simulink model "monoaxial_AZ"  (R2023b)
settings: Solver=VariableStepAuto  StartTime=0.0  StopTime=50  RelTol=1e-3
values from neighbouring files (symbols this model uses):
  meas_noise = 0.0001    [monoaxial_AZ.m]
  poles = pole(Gz)    [monoaxial_AZ.m]
  sat = 1.2    [monoaxial_AZ.m]
  Ts = 0.05    [monoaxial_AZ.m]
libraries: simulink x2, slpidlib x1
settings Model: Creator=alexz  LastModifiedBy=alexz

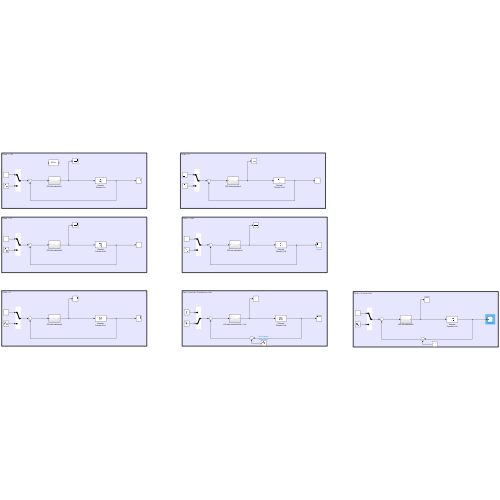
[thumbnail: Simulink's stored preview of the top-level diagram]
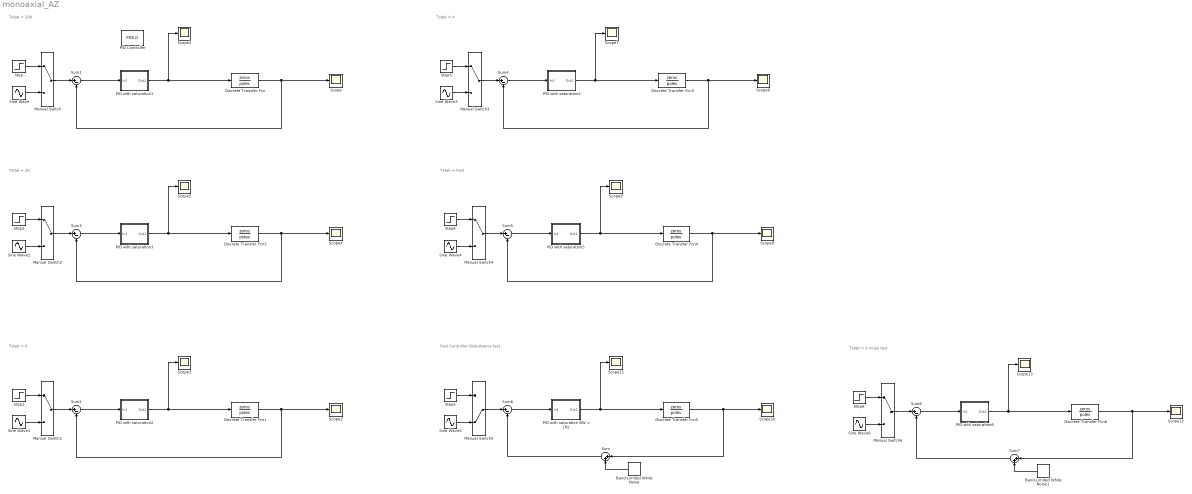
== system monoaxial_AZ ==
  note: Tstab = 100
  note: Tstab = 6
  note: Tstab = 20
  note: Tstab = 4
  note: Tstab = Fast
  note: Fast Controller Disturbance test
  note: Tstab = 4 noise test
  Band-Limited White Noise : simulink/Sources/Band-Limited White Noise  Cov=[meas_noise]  Ts=0.05  seed=[23341]
  Band-Limited White Noise1 : simulink/Sources/Band-Limited White Noise  Cov=[meas_noise]  Ts=0.05  seed=[23341]
  Discrete Transfer Fcn{,1..6} (7 alike) : DiscreteTransferFcn  Numerator=zeros  Denominator=poles
  Manual Switch{,1..4,6} (6 alike) : ManualSwitch
  Manual Switch5 : ManualSwitch  CurrentSetting=0
  PID Controller : slpidlib/PID Controller  Controller=PID  Form=Parallel  TimeDomain=Discrete-time  UseExternalTs=off  SampleTime=-1  IntegratorMethod=Forward Euler  FilterMethod=Forward Euler  ControllerParametersSource=internal  P=-0.0499947918294246  I=-1.99979167317699  UseKiTs=off  D=0  N=100  UseFilter=on  TunerSelectOption=Transfer Function Based (PID Tuner App)  InitialConditionSource=internal  InitialConditionForIntegrator=0  InitialConditionForFilter=0  DifferentiatorICPrevScaledInput=0  ExternalReset=none  TrackingMode=off  Kt=1  LimitOutput=off  SatLimitsSource=internal  UpperSaturationLimit=inf  LowerSaturationLimit=-inf  LinearizeAsGain=on  AntiWindupMode=none  Kb=1  LimitIntegrator=off  UpperIntegratorSaturationLimit=inf  LowerIntegratorSaturationLimit=-inf  POutMin=[]  POutMax=[]  IOutMin=[]  IOutMax=[]  DOutMin=[]  DOutMax=[]  NOutMin=[]  NOutMax=[]  SumOutMin=[]  SumOutMax=[]  SaturationOutMin=[]  SaturationOutMax=[]  PParamMin=[]  PParamMax=[]  IParamMin=[]  IParamMax=[]  DParamMin=[]  DParamMax=[]  NParamMin=[]  NParamMax=[]  KbParamMin=[]  KbParamMax=[]  KtParamMin=[]  KtParamMax=[]  KbOutMin=[]  KbOutMax=[]  KtOutMin=[]  KtOutMax=[]  IntegratorOutMin=[]  IntegratorOutMax=[]  FilterOutMin=[]  FilterOutMax=[]  SumI1OutMin=[]  SumI1OutMax=[]  SumI2OutMin=[]  SumI2OutMax=[]  SumI3OutMin=[]  SumI3OutMax=[]  SumI4OutMin=[]  SumI4OutMax=[]  SumDOutMin=[]  SumDOutMax=[]  DifferentiatorOutMin=[]  DifferentiatorOutMax=[]  FilterDiffOutCoefMin=[]  FilterDiffOutCoefMax=[]  ReciprocalOutMin=[]  ReciprocalOutMax=[]  SumDenOutMin=[]  SumDenOutMax=[]  SumNumOutMin=[]  SumNumOutMax=[]  DivideOutMin=[]  DivideOutMax=[]  UdiffTsProdOutMin=[]  UdiffTsProdOutMax=[]  NTsProdOutMin=[]  NTsProdOutMax=[]  UintegralTsProdOutMin=[]  UintegralTsProdOutMax=[]  UngainTsProdOutMin=[]  UngainTsProdOutMax=[]  ClampingZeroOutDataTypeStr=Inherit: Inherit via back propagation  ClampingZeroOutMin=[]  ClampingZeroOutMax=[]  FilterDenConstantOutDataTypeStr=Inherit: Inherit via back propagation  FilterDenConstantOutMin=[]  FilterDenConstantOutMax=[]  PCopyOutDataTypeStr=Inherit: Inherit via back propagation  PCopyOutMin=[]  PCopyOutMax=[]  NCopyOutDataTypeStr=Inherit: Inherit via back propagation  NCopyOutMin=[]  NCopyOutMax=[]  IntegratorContinuousStateAttributes=''  IntegratorStateMustResolveToSignalObject=off  IntegratorRTWStateStorageClass=Auto  FilterContinuousStateAttributes=''  FilterStateMustResolveToSignalObject=off  FilterRTWStateStorageClass=Auto  ParallelPVariant=InternalParameters  IdealPVariant=Disabled  IVariant=InternalParameters  DVariant=InternalParameters  IntegratorVariant=Discrete  SatVariant=Disabled  AWVariant=Passthrough  PCopyVariant=Disabled  TRVariant=Disabled  FdbkBlocksVariant=Forward  IdealPFdbkVariant=Disabled  SatFdbkVariant=Disabled  DerivativeFilterVariant=ForwardEulerFilter  NVariant=InternalParameters  NCopyVariant=Disabled  FilterICVariant=InternalICsFilter  IntegratorICVariant=InternalICs  ExternalResetVariant=Disabled  TRSumVariant=Passthrough  SumFdbkVariant=Disabled  SumVariant=Sum_PID  TsampFilterVariant=InternalTs  TsampNgainVariant=Passthrough  TsampIntegralVariant=Disabled_SignalSpec  ExternalSaturationOutDataTypeStr=Inherit: Same as second input
  PID with saturation BW = 1Hz : Subsystem
  PID with saturation1 : Subsystem
  PID with saturation2 : Subsystem
  PID with saturation3 : Subsystem
  PID with saturation4 : Subsystem
  PID with saturation5 : Subsystem
  PID with saturation6 : Subsystem
  Scope{,1..13} (14 alike) : Scope
  Sine Wave : Sin  SampleTime=0.05
  Sine Wave{1,3..6} (5 alike) : Sin  Amplitude=0.5  Frequency=0.1  SampleTime=0.05
  Sine Wave2 : Sin  SampleTime=0.05
  Step{,1..6} (7 alike) : Step  After=0.5  SampleTime=0.05
  Sum : Sum  Inputs=|++
  Sum{1..6,8} (7 alike) : Sum  Inputs=|+-
  Sum7 : Sum  Inputs=|++
  wires:
  Discrete Transfer Fcn/1 -> Sum1/2, Scope/1
  Step/1 -> Manual Switch/1
  Manual Switch/1 -> Sum1/1
  Sine Wave/1 -> Manual Switch/2
  PID with saturation1/1(Out1) -> Discrete Transfer Fcn/1, Scope1/1
  Sum1/1 -> PID with saturation1/1(In1)
  Discrete Transfer Fcn1/1 -> Sum2/2, Scope2/1
  Sine Wave1/1 -> Manual Switch1/2
  PID with saturation2/1(Out1) -> Discrete Transfer Fcn1/1, Scope3/1
  Sum2/1 -> PID with saturation2/1(In1)
  Manual Switch1/1 -> Sum2/1
  Step1/1 -> Manual Switch1/1
  Discrete Transfer Fcn2/1 -> Sum3/2, Scope4/1
  Manual Switch2/1 -> Sum3/1
  Sum3/1 -> PID with saturation3/1(In1)
  PID with saturation3/1(Out1) -> Discrete Transfer Fcn2/1, Scope5/1
  Sine Wave2/1 -> Manual Switch2/2
  Step2/1 -> Manual Switch2/1
  Discrete Transfer Fcn3/1 -> Sum4/2, Scope6/1
  Manual Switch3/1 -> Sum4/1
  Sum4/1 -> PID with saturation4/1(In1)
  PID with saturation4/1(Out1) -> Discrete Transfer Fcn3/1, Scope7/1
  Sine Wave3/1 -> Manual Switch3/2
  Step3/1 -> Manual Switch3/1
  Sine Wave4/1 -> Manual Switch4/2
  Step4/1 -> Manual Switch4/1
  PID with saturation5/1(Out1) -> Discrete Transfer Fcn4/1, Scope9/1
  Discrete Transfer Fcn4/1 -> Sum5/2, Scope8/1
  Sum5/1 -> PID with saturation5/1(In1)
  Manual Switch4/1 -> Sum5/1
  Sum6/1 -> PID with saturation BW = 1Hz/1(In1)
  Manual Switch5/1 -> Sum6/1
  PID with saturation BW = 1Hz/1(Out1) -> Discrete Transfer Fcn5/1, Scope11/1
  Sine Wave5/1 -> Manual Switch5/2
  Discrete Transfer Fcn5/1 -> Sum/1, Scope10/1
  Step5/1 -> Manual Switch5/1
  Sum/1 -> Sum6/2
  Band-Limited White Noise/1 -> Sum/2
  Step6/1 -> Manual Switch6/1
  Discrete Transfer Fcn6/1 -> Sum7/1, Scope12/1
  Sine Wave6/1 -> Manual Switch6/2
  Sum8/1 -> PID with saturation6/1(In1)
  Band-Limited White Noise1/1 -> Sum7/2
  Manual Switch6/1 -> Sum8/1
  Sum7/1 -> Sum8/2
  PID with saturation6/1(Out1) -> Discrete Transfer Fcn6/1, Scope13/1

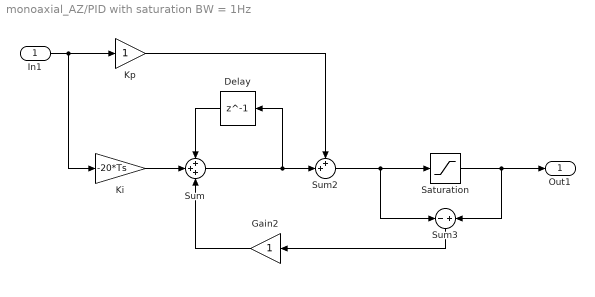
== system monoaxial_AZ/PID with saturation BW = 1Hz ==
  In1 : Inport
  Delay : Delay  DelayLength=1
  Gain2 : Gain
  Ki : Gain  Gain=-20*Ts
  Kp : Gain
  Saturation : Saturate  UpperLimit=sat  LowerLimit=-sat
  Sum : Sum  Inputs=+++
  Sum2 : Sum  Inputs=++|
  Sum3 : Sum  Inputs=-+
  Out1 : Outport
  wires:
  In1/1 -> Ki/1, Kp/1
  Sum2/1 -> Sum3/1, Saturation/1
  Sum3/1 -> Gain2/1
  Saturation/1 -> Out1/1, Sum3/2
  Kp/1 -> Sum2/1
  Sum/1 -> Sum2/2, Delay/1
  Gain2/1 -> Sum/3
  Ki/1 -> Sum/2
  Delay/1 -> Sum/1

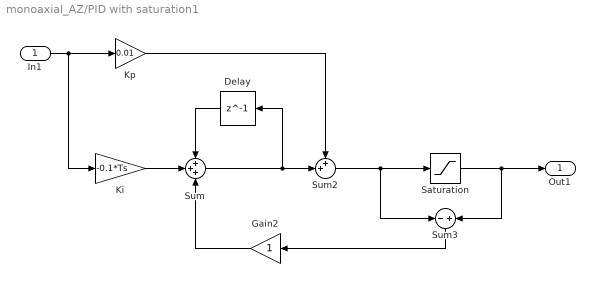
== system monoaxial_AZ/PID with saturation1 ==
  In1 : Inport
  Delay : Delay  DelayLength=1
  Gain2 : Gain
  Ki : Gain  Gain=-0.1*Ts
  Kp : Gain  Gain=0.01
  Saturation : Saturate  UpperLimit=sat  LowerLimit=-sat
  Sum : Sum  Inputs=+++
  Sum2 : Sum  Inputs=++|
  Sum3 : Sum  Inputs=-+
  Out1 : Outport
  wires:
  In1/1 -> Ki/1, Kp/1
  Sum2/1 -> Sum3/1, Saturation/1
  Sum3/1 -> Gain2/1
  Saturation/1 -> Out1/1, Sum3/2
  Kp/1 -> Sum2/1
  Sum/1 -> Sum2/2, Delay/1
  Gain2/1 -> Sum/3
  Ki/1 -> Sum/2
  Delay/1 -> Sum/1

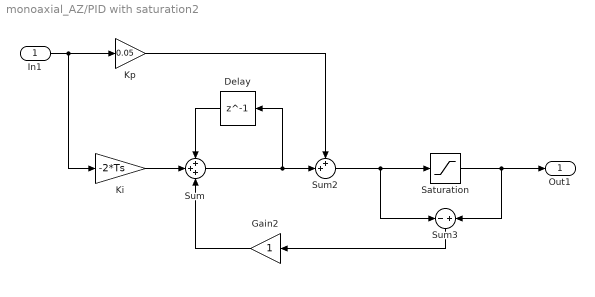
== system monoaxial_AZ/PID with saturation2 ==
  In1 : Inport
  Delay : Delay  DelayLength=1
  Gain2 : Gain
  Ki : Gain  Gain=-2*Ts
  Kp : Gain  Gain=0.05
  Saturation : Saturate  UpperLimit=sat  LowerLimit=-sat
  Sum : Sum  Inputs=+++
  Sum2 : Sum  Inputs=++|
  Sum3 : Sum  Inputs=-+
  Out1 : Outport
  wires:
  In1/1 -> Ki/1, Kp/1
  Sum2/1 -> Sum3/1, Saturation/1
  Sum3/1 -> Gain2/1
  Saturation/1 -> Out1/1, Sum3/2
  Kp/1 -> Sum2/1
  Sum/1 -> Sum2/2, Delay/1
  Gain2/1 -> Sum/3
  Ki/1 -> Sum/2
  Delay/1 -> Sum/1

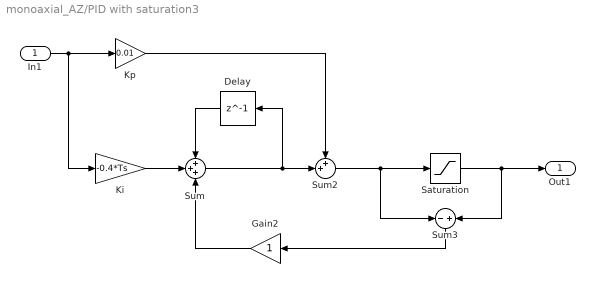
== system monoaxial_AZ/PID with saturation3 ==
  In1 : Inport
  Delay : Delay  DelayLength=1
  Gain2 : Gain
  Ki : Gain  Gain=-0.4*Ts
  Kp : Gain  Gain=0.01
  Saturation : Saturate  UpperLimit=sat  LowerLimit=-sat
  Sum : Sum  Inputs=+++
  Sum2 : Sum  Inputs=++|
  Sum3 : Sum  Inputs=-+
  Out1 : Outport
  wires:
  In1/1 -> Ki/1, Kp/1
  Sum2/1 -> Sum3/1, Saturation/1
  Sum3/1 -> Gain2/1
  Saturation/1 -> Out1/1, Sum3/2
  Kp/1 -> Sum2/1
  Sum/1 -> Sum2/2, Delay/1
  Gain2/1 -> Sum/3
  Ki/1 -> Sum/2
  Delay/1 -> Sum/1

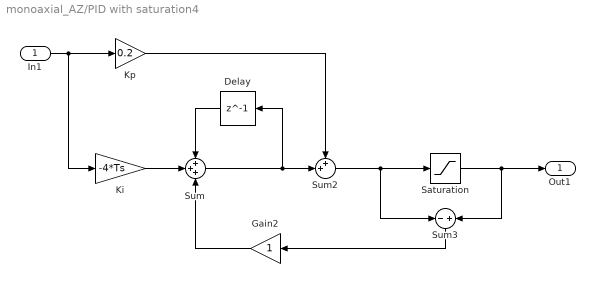
== system monoaxial_AZ/PID with saturation4 ==
  In1 : Inport
  Delay : Delay  DelayLength=1
  Gain2 : Gain
  Ki : Gain  Gain=-4*Ts
  Kp : Gain  Gain=0.2
  Saturation : Saturate  UpperLimit=sat  LowerLimit=-sat
  Sum : Sum  Inputs=+++
  Sum2 : Sum  Inputs=++|
  Sum3 : Sum  Inputs=-+
  Out1 : Outport
  wires:
  In1/1 -> Ki/1, Kp/1
  Sum2/1 -> Sum3/1, Saturation/1
  Sum3/1 -> Gain2/1
  Saturation/1 -> Out1/1, Sum3/2
  Kp/1 -> Sum2/1
  Sum/1 -> Sum2/2, Delay/1
  Gain2/1 -> Sum/3
  Ki/1 -> Sum/2
  Delay/1 -> Sum/1

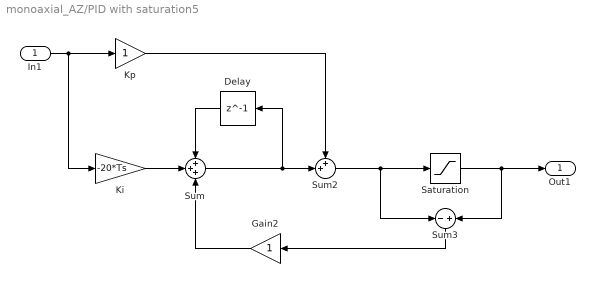
== system monoaxial_AZ/PID with saturation5 ==
  In1 : Inport
  Delay : Delay  DelayLength=1
  Gain2 : Gain
  Ki : Gain  Gain=-20*Ts
  Kp : Gain
  Saturation : Saturate  UpperLimit=sat  LowerLimit=-sat
  Sum : Sum  Inputs=+++
  Sum2 : Sum  Inputs=++|
  Sum3 : Sum  Inputs=-+
  Out1 : Outport
  wires:
  In1/1 -> Ki/1, Kp/1
  Sum2/1 -> Sum3/1, Saturation/1
  Sum3/1 -> Gain2/1
  Saturation/1 -> Out1/1, Sum3/2
  Kp/1 -> Sum2/1
  Sum/1 -> Sum2/2, Delay/1
  Gain2/1 -> Sum/3
  Ki/1 -> Sum/2
  Delay/1 -> Sum/1

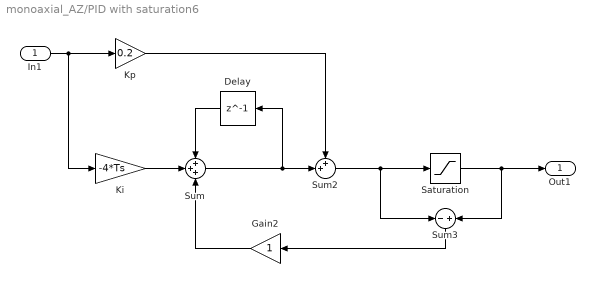
== system monoaxial_AZ/PID with saturation6 ==
  In1 : Inport
  Delay : Delay  DelayLength=1
  Gain2 : Gain
  Ki : Gain  Gain=-4*Ts
  Kp : Gain  Gain=0.2
  Saturation : Saturate  UpperLimit=sat  LowerLimit=-sat
  Sum : Sum  Inputs=+++
  Sum2 : Sum  Inputs=++|
  Sum3 : Sum  Inputs=-+
  Out1 : Outport
  wires:
  In1/1 -> Ki/1, Kp/1
  Sum2/1 -> Sum3/1, Saturation/1
  Sum3/1 -> Gain2/1
  Saturation/1 -> Out1/1, Sum3/2
  Kp/1 -> Sum2/1
  Sum/1 -> Sum2/2, Delay/1
  Gain2/1 -> Sum/3
  Ki/1 -> Sum/2
  Delay/1 -> Sum/1
